simulink library "mobileRoboticsLib"  (R2017b)
settings: Solver=VariableStepAuto  StartTime=0.0  StopTime=10.0  RelTol=1e-3
undefined symbols (not defined in the file): b, DiscIntNeverNeededParam, r, X, Y, Z
libraries: sm_lib x67, nesl_utility x25, mobileRoboticsLib x11
(part 4 of 4)

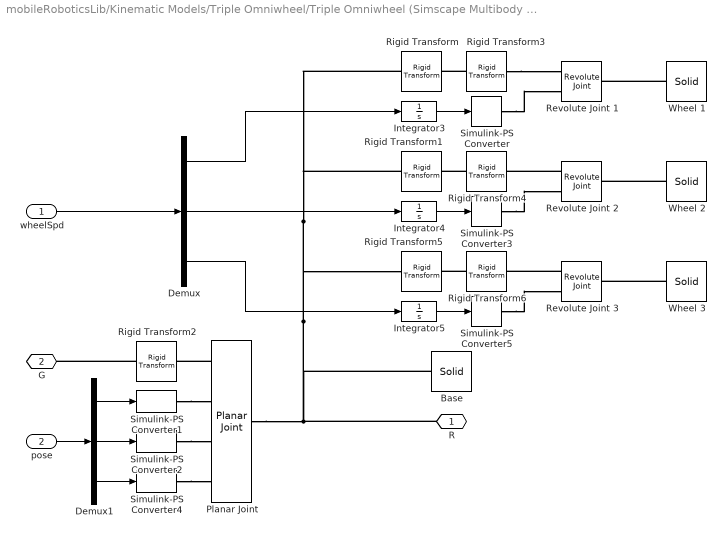
== system mobileRoboticsLib/Kinematic Models/Triple Omniwheel/Triple Omniwheel (Simscape Multibody Model) ==
  wheelSpd : Inport
  pose : Inport  Port=2
  Base : sm_lib/Body Elements/Solid  InertiaType=CalculateFromGeometry  Mass=chassisMass  MassUnits=kg  CenterOfMass=[0 0 0]  CenterOfMassUnits=m  MomentsOfInertia=[1 1 1]  MomentsOfInertiaUnits=kg*m^2  ProductsOfInertia=[1 1 1]  ProductsOfInertiaUnits=kg*m^2  DensityBased=on  Density=chassisMass  DensityUnits=kg/m^3  DoExposeReferenceFrame=on  SerializedFrames=<Frames/>  GraphicType=FromGeometry  MarkerShape=Sphere  MarkerSize=10  GraphicVisPropType=SimpleVisualProperties  GraphicDiffuseColor=chassisColor  GraphicSpecularColor=[0.5 0.5 0.5 1.0]  GraphicAmbientColor=[0.15 0.15 0.15 1.0]  GraphicEmissiveColor=[0.0 0.0 0.0 1.0]  GraphicShininess=75  GraphicOpacity=1.0  GeometryShape=Cylinder  RectangleSize=[1 1]  RectangleSizeUnits=m  BrickDimensions=[1 1 1]  BrickDimensionUnits=m  CylinderRadius=robotRadius-(wheelThickness/2)  CylinderRadiusUnits=m  CylinderLength=chassisThickness  CylinderLengthUnits=m  SphereRadius=1  SphereRadiusUnits=m  EllipsoidRadii=[1 1 1]  EllipsoidRadiiUnits=m  ExtrusionCrossSection=[1 1; -1 1; -1 -1; 1 -1]  ExtrusionCrossSectionUnits=m  ExtrusionLength=1  ExtrusionLengthUnits=m  PolygonNumSides=3  PolygonOuterRadius=1  PolygonOuterRadiusUnits=m  ExtGeomFileType=STEP  ExtGeomFileUnits=m  RevolutionCrossSection=[1 1; 1 -1; 2 -1; 2 1]  RevolutionCrossSectionUnits=m  RevolutionExtent=Full  RevolutionAngle=180  RevolutionAngleUnits=deg
  Demux : Demux  Outputs=3
  Demux1 : Demux  Outputs=3
  Integrator3 : Integrator
  Integrator4 : Integrator
  Integrator5 : Integrator
  Planar Joint : sm_lib/Joints/Planar Joint  SenseConstraintForce=off  SenseConstraintForceX=off  SenseConstraintForceY=off  SenseConstraintForceZ=off  SenseConstraintTorque=off  SenseConstraintTorqueX=off  SenseConstraintTorqueY=off  SenseConstraintTorqueZ=off  SenseTotalForce=off  SenseTotalForceX=off  SenseTotalForceY=off  SenseTotalForceZ=off  SenseTotalTorque=off  SenseTotalTorqueX=off  SenseTotalTorqueY=off  SenseTotalTorqueZ=off  CompositeWrenchDir=FollowerOnBase  CompositeWrenchFrame=BaseFrame  PxEquilibriumPosition=0  PxEquilibriumPositionUnits=m  PxSpringStiffness=0  PxSpringStiffnessUnits=N/m  PxDampingCoefficient=0  PxDampingCoefficientUnits=N/(m/s)  PxTorqueActuationMode=ComputedTorque  PxMotionActuationMode=InputMotion  PxSensePosition=off  PxSenseVelocity=off  PxSenseAcceleration=off  PxSenseTorqueForce=off  PxPositionTargetSpecify=on  PxPositionTargetPriority=High  PxPositionTargetValue=initX  PxPositionTargetValueUnits=m  PxVelocityTargetSpecify=off  PxVelocityTargetPriority=High  PxVelocityTargetValue=0  PxVelocityTargetValueUnits=m/s  PyEquilibriumPosition=0  PyEquilibriumPositionUnits=m  PySpringStiffness=0  PySpringStiffnessUnits=N/m  PyDampingCoefficient=0  PyDampingCoefficientUnits=N/(m/s)  PyTorqueActuationMode=ComputedTorque  PyMotionActuationMode=InputMotion  PySensePosition=off  PySenseVelocity=off  PySenseAcceleration=off  PySenseTorqueForce=off  PyPositionTargetSpecify=on  PyPositionTargetPriority=High  PyPositionTargetValue=initY  PyPositionTargetValueUnits=m  PyVelocityTargetSpecify=off  PyVelocityTargetPriority=High  PyVelocityTargetValue=0  PyVelocityTargetValueUnits=m/s  RzEquilibriumPosition=0  RzEquilibriumPositionUnits=deg  RzSpringStiffness=0  RzSpringStiffnessUnits=N*m/deg  RzDampingCoefficient=0  RzDampingCoefficientUnits=N*m/(deg/s)  RzTorqueActuationMode=ComputedTorque  RzMotionActuationMode=InputMotion  RzSensePosition=off  RzSenseVelocity=off  RzSenseAcceleration=off  RzSenseTorqueForce=off  RzPositionTargetSpecify=on  RzPositionTargetPriority=High  RzPositionTargetValue=initAngle  RzPositionTargetValueUnits=rad  RzVelocityTargetSpecify=off  RzVelocityTargetPriority=High  RzVelocityTargetValue=0  RzVelocityTargetValueUnits=deg/s
  Revolute Joint 1 : sm_lib/Joints/Revolute Joint  SenseConstraintForce=off  SenseConstraintForceX=off  SenseConstraintForceY=off  SenseConstraintForceZ=off  SenseConstraintTorque=off  SenseConstraintTorqueX=off  SenseConstraintTorqueY=off  SenseConstraintTorqueZ=off  SenseTotalForce=off  SenseTotalForceX=off  SenseTotalForceY=off  SenseTotalForceZ=off  SenseTotalTorque=off  SenseTotalTorqueX=off  SenseTotalTorqueY=off  SenseTotalTorqueZ=off  CompositeWrenchDir=FollowerOnBase  CompositeWrenchFrame=BaseFrame  EquilibriumPosition=0  EquilibriumPositionUnits=deg  SpringStiffness=0  SpringStiffnessUnits=N*m/deg  DampingCoefficient=0  DampingCoefficientUnits=N*m/(deg/s)  TorqueActuationMode=ComputedTorque  MotionActuationMode=InputMotion  SensePosition=off  SenseVelocity=off  SenseAcceleration=off  SenseTorqueForce=off  PositionTargetSpecify=off  PositionTargetPriority=High  PositionTargetValue=0  PositionTargetValueUnits=deg  VelocityTargetSpecify=off  VelocityTargetPriority=High  VelocityTargetValue=0  VelocityTargetValueUnits=deg/s
  Revolute Joint 2 : sm_lib/Joints/Revolute Joint  SenseConstraintForce=off  SenseConstraintForceX=off  SenseConstraintForceY=off  SenseConstraintForceZ=off  SenseConstraintTorque=off  SenseConstraintTorqueX=off  SenseConstraintTorqueY=off  SenseConstraintTorqueZ=off  SenseTotalForce=off  SenseTotalForceX=off  SenseTotalForceY=off  SenseTotalForceZ=off  SenseTotalTorque=off  SenseTotalTorqueX=off  SenseTotalTorqueY=off  SenseTotalTorqueZ=off  CompositeWrenchDir=FollowerOnBase  CompositeWrenchFrame=BaseFrame  EquilibriumPosition=0  EquilibriumPositionUnits=deg  SpringStiffness=0  SpringStiffnessUnits=N*m/deg  DampingCoefficient=0  DampingCoefficientUnits=N*m/(deg/s)  TorqueActuationMode=ComputedTorque  MotionActuationMode=InputMotion  SensePosition=off  SenseVelocity=off  SenseAcceleration=off  SenseTorqueForce=off  PositionTargetSpecify=off  PositionTargetPriority=High  PositionTargetValue=0  PositionTargetValueUnits=deg  VelocityTargetSpecify=off  VelocityTargetPriority=High  VelocityTargetValue=0  VelocityTargetValueUnits=deg/s
  Revolute Joint 3 : sm_lib/Joints/Revolute Joint  SenseConstraintForce=off  SenseConstraintForceX=off  SenseConstraintForceY=off  SenseConstraintForceZ=off  SenseConstraintTorque=off  SenseConstraintTorqueX=off  SenseConstraintTorqueY=off  SenseConstraintTorqueZ=off  SenseTotalForce=off  SenseTotalForceX=off  SenseTotalForceY=off  SenseTotalForceZ=off  SenseTotalTorque=off  SenseTotalTorqueX=off  SenseTotalTorqueY=off  SenseTotalTorqueZ=off  CompositeWrenchDir=FollowerOnBase  CompositeWrenchFrame=BaseFrame  EquilibriumPosition=0  EquilibriumPositionUnits=deg  SpringStiffness=0  SpringStiffnessUnits=N*m/deg  DampingCoefficient=0  DampingCoefficientUnits=N*m/(deg/s)  TorqueActuationMode=ComputedTorque  MotionActuationMode=InputMotion  SensePosition=off  SenseVelocity=off  SenseAcceleration=off  SenseTorqueForce=off  PositionTargetSpecify=off  PositionTargetPriority=High  PositionTargetValue=0  PositionTargetValueUnits=deg  VelocityTargetSpecify=off  VelocityTargetPriority=High  VelocityTargetValue=0  VelocityTargetValueUnits=deg/s
  Rigid Transform : sm_lib/Frames and Transforms/Rigid Transform  TranslationMethod=Cartesian  TranslationStandardOffset=0  TranslationLengthUnit=m  TranslationStandardAxis=+Y  TranslationCartesianOffset=[robotRadius*cos(wheelAngles(1)) robotRadius*sin(wheelAngles(1)) 0]  TranslationROffset=0  TranslationROffsetUnits=m  TranslationZOffset=0  TranslationZOffsetUnits=m  TranslationThetaOffset=0  TranslationThetaOffsetUnits=deg  RotationMethod=AlignedAxes  RotationAngleUnits=deg  RotationStandardAxis=+Z  RotationAngle=0.0  RotationArbitraryAxis=[0 0 1]  FollAlignAxisA=+Z  BaseAlignAxisA=+Y  FollAlignAxisB=+X  BaseAlignAxisB=+X  RotationSequenceAxes=FollowerAxes  RotationSequence=XYX  RotationSequenceAngles=[0 0 0]  RotationSequenceAnglesUnits=deg  RotationMatrix=[1 0 0; 0 1 0; 0 0 1]
  Rigid Transform1 : sm_lib/Frames and Transforms/Rigid Transform  TranslationMethod=Cartesian  TranslationStandardOffset=0  TranslationLengthUnit=m  TranslationStandardAxis=+Y  TranslationCartesianOffset=[robotRadius*cos(wheelAngles(2)) robotRadius*sin(wheelAngles(2)) 0]  TranslationROffset=0  TranslationROffsetUnits=m  TranslationZOffset=0  TranslationZOffsetUnits=m  TranslationThetaOffset=0  TranslationThetaOffsetUnits=deg  RotationMethod=AlignedAxes  RotationAngleUnits=deg  RotationStandardAxis=+Z  RotationAngle=0.0  RotationArbitraryAxis=[0 0 1]  FollAlignAxisA=+Z  BaseAlignAxisA=+Y  FollAlignAxisB=+X  BaseAlignAxisB=+X  RotationSequenceAxes=FollowerAxes  RotationSequence=XYX  RotationSequenceAngles=[0 0 0]  RotationSequenceAnglesUnits=deg  RotationMatrix=[1 0 0; 0 1 0; 0 0 1]
  Rigid Transform2 : sm_lib/Frames and Transforms/Rigid Transform  TranslationMethod=StandardAxis  TranslationStandardOffset=wheelRadius  TranslationLengthUnit=m  TranslationStandardAxis=+Z  TranslationCartesianOffset=[0 0 0]  TranslationROffset=0  TranslationROffsetUnits=m  TranslationZOffset=0  TranslationZOffsetUnits=m  TranslationThetaOffset=0  TranslationThetaOffsetUnits=deg  RotationMethod=None  RotationAngleUnits=deg  RotationStandardAxis=+Z  RotationAngle=0.0  RotationArbitraryAxis=[0 0 1]  FollAlignAxisA=+Z  BaseAlignAxisA=+Y  FollAlignAxisB=+X  BaseAlignAxisB=+X  RotationSequenceAxes=FollowerAxes  RotationSequence=XYX  RotationSequenceAngles=[0 0 0]  RotationSequenceAnglesUnits=deg  RotationMatrix=[1 0 0; 0 1 0; 0 0 1]
  Rigid Transform3 : sm_lib/Frames and Transforms/Rigid Transform  TranslationMethod=None  TranslationStandardOffset=0  TranslationLengthUnit=m  TranslationStandardAxis=+Z  TranslationCartesianOffset=[0 0 0]  TranslationROffset=0  TranslationROffsetUnits=m  TranslationZOffset=0  TranslationZOffsetUnits=m  TranslationThetaOffset=0  TranslationThetaOffsetUnits=deg  RotationMethod=StandardAxis  RotationAngleUnits=rad  RotationStandardAxis=+Y  RotationAngle=pi/2-wheelAngles(1)  RotationArbitraryAxis=[0 0 1]  FollAlignAxisA=+X  BaseAlignAxisA=+Y  FollAlignAxisB=+Y  BaseAlignAxisB=+Z  RotationSequenceAxes=FollowerAxes  RotationSequence=XYX  RotationSequenceAngles=[0 0 0]  RotationSequenceAnglesUnits=deg  RotationMatrix=[1 0 0; 0 1 0; 0 0 1]
  Rigid Transform4 : sm_lib/Frames and Transforms/Rigid Transform  TranslationMethod=None  TranslationStandardOffset=0  TranslationLengthUnit=m  TranslationStandardAxis=+Z  TranslationCartesianOffset=[0 0 0]  TranslationROffset=0  TranslationROffsetUnits=m  TranslationZOffset=0  TranslationZOffsetUnits=m  TranslationThetaOffset=0  TranslationThetaOffsetUnits=deg  RotationMethod=StandardAxis  RotationAngleUnits=rad  RotationStandardAxis=+Y  RotationAngle=pi/2-wheelAngles(2)  RotationArbitraryAxis=[0 0 1]  FollAlignAxisA=+X  BaseAlignAxisA=+Y  FollAlignAxisB=+Y  BaseAlignAxisB=+Z  RotationSequenceAxes=FollowerAxes  RotationSequence=XYX  RotationSequenceAngles=[0 0 0]  RotationSequenceAnglesUnits=deg  RotationMatrix=[1 0 0; 0 1 0; 0 0 1]
  Rigid Transform5 : sm_lib/Frames and Transforms/Rigid Transform  TranslationMethod=Cartesian  TranslationStandardOffset=0  TranslationLengthUnit=m  TranslationStandardAxis=+Y  TranslationCartesianOffset=[robotRadius*cos(wheelAngles(3)) robotRadius*sin(wheelAngles(3)) 0]  TranslationROffset=0  TranslationROffsetUnits=m  TranslationZOffset=0  TranslationZOffsetUnits=m  TranslationThetaOffset=0  TranslationThetaOffsetUnits=deg  RotationMethod=AlignedAxes  RotationAngleUnits=deg  RotationStandardAxis=+Z  RotationAngle=0.0  RotationArbitraryAxis=[0 0 1]  FollAlignAxisA=+Z  BaseAlignAxisA=+Y  FollAlignAxisB=+X  BaseAlignAxisB=+X  RotationSequenceAxes=FollowerAxes  RotationSequence=XYX  RotationSequenceAngles=[0 0 0]  RotationSequenceAnglesUnits=deg  RotationMatrix=[1 0 0; 0 1 0; 0 0 1]
  Rigid Transform6 : sm_lib/Frames and Transforms/Rigid Transform  TranslationMethod=None  TranslationStandardOffset=0  TranslationLengthUnit=m  TranslationStandardAxis=+Z  TranslationCartesianOffset=[0 0 0]  TranslationROffset=0  TranslationROffsetUnits=m  TranslationZOffset=0  TranslationZOffsetUnits=m  TranslationThetaOffset=0  TranslationThetaOffsetUnits=deg  RotationMethod=StandardAxis  RotationAngleUnits=rad  RotationStandardAxis=+Y  RotationAngle=pi/2-wheelAngles(3)  RotationArbitraryAxis=[0 0 1]  FollAlignAxisA=+X  BaseAlignAxisA=+Y  FollAlignAxisB=+Y  BaseAlignAxisB=+Z  RotationSequenceAxes=FollowerAxes  RotationSequence=XYX  RotationSequenceAngles=[0 0 0]  RotationSequenceAnglesUnits=deg  RotationMatrix=[1 0 0; 0 1 0; 0 0 1]
  Simulink-PS Converter{,1..5} (6 alike) : nesl_utility/Simulink-PS Converter  PhysicalDomain=network_engine_domain  SubClassName=ps_input  LeftPortType=input  RightPortType=output  PseudoPeriodic=off  Frequencies=[]  NoiseDistribution=none  NoiseParameters=[]  Unit=1  AffineConversion=off  FilteringAndDerivatives=filter  SimscapeFilterOrder=2  InputFilterTimeConstant=timeConstant  UdotUserProvided=0
  Wheel 1 : sm_lib/Body Elements/Solid  InertiaType=CalculateFromGeometry  Mass=wheelMass  MassUnits=kg  CenterOfMass=[0 0 0]  CenterOfMassUnits=m  MomentsOfInertia=[1 1 1]  MomentsOfInertiaUnits=kg*m^2  ProductsOfInertia=[1 1 1]  ProductsOfInertiaUnits=kg*m^2  DensityBased=on  Density=1000  DensityUnits=kg/m^3  DoExposeReferenceFrame=on  SerializedFrames=<Frames/>  GraphicType=FromGeometry  MarkerShape=Sphere  MarkerSize=10  GraphicVisPropType=SimpleVisualProperties  GraphicDiffuseColor=wheelColor  GraphicSpecularColor=[0.5 0.5 0.5 1.0]  GraphicAmbientColor=[0.15 0.15 0.15 1.0]  GraphicEmissiveColor=[0.0 0.0 0.0 1.0]  GraphicShininess=75  GraphicOpacity=1.0  GeometryShape=Cylinder  RectangleSize=[1 1]  RectangleSizeUnits=m  BrickDimensions=[1 1 1]  BrickDimensionUnits=m  CylinderRadius=wheelRadius  CylinderRadiusUnits=m  CylinderLength=wheelThickness  CylinderLengthUnits=m  SphereRadius=1  SphereRadiusUnits=m  EllipsoidRadii=[1 1 1]  EllipsoidRadiiUnits=m  ExtrusionCrossSection=[1 1; -1 1; -1 -1; 1 -1]  ExtrusionCrossSectionUnits=m  ExtrusionLength=1  ExtrusionLengthUnits=m  PolygonNumSides=3  PolygonOuterRadius=1  PolygonOuterRadiusUnits=m  ExtGeomFileType=STEP  ExtGeomFileUnits=m  RevolutionCrossSection=[1 1; 1 -1; 2 -1; 2 1]  RevolutionCrossSectionUnits=m  RevolutionExtent=Full  RevolutionAngle=180  RevolutionAngleUnits=deg
  Wheel 2 : sm_lib/Body Elements/Solid  InertiaType=CalculateFromGeometry  Mass=wheelMass  MassUnits=kg  CenterOfMass=[0 0 0]  CenterOfMassUnits=m  MomentsOfInertia=[1 1 1]  MomentsOfInertiaUnits=kg*m^2  ProductsOfInertia=[1 1 1]  ProductsOfInertiaUnits=kg*m^2  DensityBased=on  Density=1000  DensityUnits=kg/m^3  DoExposeReferenceFrame=on  SerializedFrames=<Frames/>  GraphicType=FromGeometry  MarkerShape=Sphere  MarkerSize=10  GraphicVisPropType=SimpleVisualProperties  GraphicDiffuseColor=wheelColor  GraphicSpecularColor=[0.5 0.5 0.5 1.0]  GraphicAmbientColor=[0.15 0.15 0.15 1.0]  GraphicEmissiveColor=[0.0 0.0 0.0 1.0]  GraphicShininess=75  GraphicOpacity=1.0  GeometryShape=Cylinder  RectangleSize=[1 1]  RectangleSizeUnits=m  BrickDimensions=[1 1 1]  BrickDimensionUnits=m  CylinderRadius=wheelRadius  CylinderRadiusUnits=m  CylinderLength=wheelThickness  CylinderLengthUnits=m  SphereRadius=1  SphereRadiusUnits=m  EllipsoidRadii=[1 1 1]  EllipsoidRadiiUnits=m  ExtrusionCrossSection=[1 1; -1 1; -1 -1; 1 -1]  ExtrusionCrossSectionUnits=m  ExtrusionLength=1  ExtrusionLengthUnits=m  PolygonNumSides=3  PolygonOuterRadius=1  PolygonOuterRadiusUnits=m  ExtGeomFileType=STEP  ExtGeomFileUnits=m  RevolutionCrossSection=[1 1; 1 -1; 2 -1; 2 1]  RevolutionCrossSectionUnits=m  RevolutionExtent=Full  RevolutionAngle=180  RevolutionAngleUnits=deg
  Wheel 3 : sm_lib/Body Elements/Solid  InertiaType=CalculateFromGeometry  Mass=wheelMass  MassUnits=kg  CenterOfMass=[0 0 0]  CenterOfMassUnits=m  MomentsOfInertia=[1 1 1]  MomentsOfInertiaUnits=kg*m^2  ProductsOfInertia=[1 1 1]  ProductsOfInertiaUnits=kg*m^2  DensityBased=on  Density=1000  DensityUnits=kg/m^3  DoExposeReferenceFrame=on  SerializedFrames=<Frames/>  GraphicType=FromGeometry  MarkerShape=Sphere  MarkerSize=10  GraphicVisPropType=SimpleVisualProperties  GraphicDiffuseColor=wheelColor  GraphicSpecularColor=[0.5 0.5 0.5 1.0]  GraphicAmbientColor=[0.15 0.15 0.15 1.0]  GraphicEmissiveColor=[0.0 0.0 0.0 1.0]  GraphicShininess=75  GraphicOpacity=1.0  GeometryShape=Cylinder  RectangleSize=[1 1]  RectangleSizeUnits=m  BrickDimensions=[1 1 1]  BrickDimensionUnits=m  CylinderRadius=wheelRadius  CylinderRadiusUnits=m  CylinderLength=wheelThickness  CylinderLengthUnits=m  SphereRadius=1  SphereRadiusUnits=m  EllipsoidRadii=[1 1 1]  EllipsoidRadiiUnits=m  ExtrusionCrossSection=[1 1; -1 1; -1 -1; 1 -1]  ExtrusionCrossSectionUnits=m  ExtrusionLength=1  ExtrusionLengthUnits=m  PolygonNumSides=3  PolygonOuterRadius=1  PolygonOuterRadiusUnits=m  ExtGeomFileType=STEP  ExtGeomFileUnits=m  RevolutionCrossSection=[1 1; 1 -1; 2 -1; 2 1]  RevolutionCrossSectionUnits=m  RevolutionExtent=Full  RevolutionAngle=180  RevolutionAngleUnits=deg
  R : PMIOPort  Port=1  Side=Right
  G : PMIOPort  Port=2  Side=Right
  wires:
  wheelSpd/1 -> Demux/1
  Demux1/1 -> Simulink-PS Converter1/1
  Demux1/2 -> Simulink-PS Converter2/1
  Demux1/3 -> Simulink-PS Converter4/1
  pose/1 -> Demux1/1
  Integrator5/1 -> Simulink-PS Converter5/1
  Integrator3/1 -> Simulink-PS Converter/1
  Integrator4/1 -> Simulink-PS Converter3/1
  Demux/1 -> Integrator3/1
  Demux/2 -> Integrator4/1
  Demux/3 -> Integrator5/1
  connections:
  Simulink-PS Converter1/RConn1 -- Planar Joint/LConn2
  Rigid Transform2/LConn1 -- G/RConn1
  Simulink-PS Converter4/RConn1 -- Planar Joint/LConn4
  Simulink-PS Converter2/RConn1 -- Planar Joint/LConn3
  Planar Joint/LConn1 -- Rigid Transform2/RConn1
  R/RConn1 -- Planar Joint/RConn1 -- Base/RConn1 -- Rigid Transform/LConn1 -- Rigid Transform1/LConn1 -- Rigid Transform5/LConn1
  Rigid Transform6/LConn1 -- Rigid Transform5/RConn1
  Rigid Transform3/RConn1 -- Revolute Joint 1/LConn1
  Revolute Joint 3/LConn1 -- Rigid Transform6/RConn1
  Revolute Joint 2/LConn1 -- Rigid Transform4/RConn1
  Simulink-PS Converter3/RConn1 -- Revolute Joint 2/LConn2
  Simulink-PS Converter5/RConn1 -- Revolute Joint 3/LConn2
  Wheel 1/RConn1 -- Revolute Joint 1/RConn1
  Rigid Transform3/LConn1 -- Rigid Transform/RConn1
  Simulink-PS Converter/RConn1 -- Revolute Joint 1/LConn2
  Wheel 2/RConn1 -- Revolute Joint 2/RConn1
  Rigid Transform4/LConn1 -- Rigid Transform1/RConn1
  Wheel 3/RConn1 -- Revolute Joint 3/RConn1

== system mobileRoboticsLib/Kinematic Models/Triple Omniwheel/Triple Omniwheel Forward Kinematics ==
  wheelSpd : Inport
  MATLAB Function : MATLAB Function  TreatAsAtomicUnit=on
  bodySpd : Outport
  wires:
  wheelSpd/1 -> MATLAB Function/1(wheelSpeeds)  "wheelSpeeds"
  MATLAB Function/1(bodySpeed) -> bodySpd/1  "bodySpeed"

== system mobileRoboticsLib/Kinematic Models/Triple Omniwheel/Triple Omniwheel Inverse Kinematics  ==
  vRef : Inport
  MATLAB Function : MATLAB Function  TreatAsAtomicUnit=on
  wheelSpd : Outport
  wires:
  MATLAB Function/1(wheelSpeeds) -> wheelSpd/1  "wheelSpeeds"
  vRef/1 -> MATLAB Function/1(bodySpeed)  "bodySpeed"

== system mobileRoboticsLib/Kinematic Models/Triple Omniwheel/Triple Omniwheel Simulation ==
  wheelSpd : Inport
  Generic Robot Simulation : mobileRoboticsLib/Utilities/Generic Vehicle Simulation  initX=initX  initY=initY  initAngle=initAngle  Ts=Ts
      settings: SourceProductName=Mobile Robotics Simulation Toolbox
  Triple Omniwheel Forward Kinematics : mobileRoboticsLib/Kinematic Models/Triple Omniwheel/Triple Omniwheel Forward Kinematics  wheelRadius=wheelRadius  robotRadius=robotRadius  wheelAngles=wheelAngles
      settings: SourceProductName=Mobile Robotics Simulation Toolbox
  pose : Outport
  wires:
  wheelSpd/1 -> Triple Omniwheel Forward Kinematics/1
  Triple Omniwheel Forward Kinematics/1 -> Generic Robot Simulation/1
  Generic Robot Simulation/1 -> pose/1

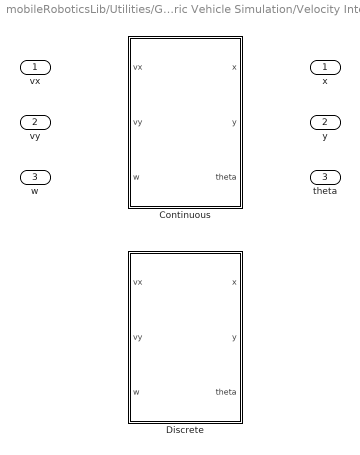
== system mobileRoboticsLib/Utilities/Generic Vehicle Simulation/Velocity Integrator ==
  "vx " : Inport
  "vy " : Inport  Port=2
  "w " : Inport  Port=3
  Continuous : Subsystem  VariantControl=mode==1
  Discrete : Subsystem  VariantControl=mode==2
  " x" : Outport
  " y" : Outport  Port=2
  " theta" : Outport  Port=3

== system mobileRoboticsLib/Kinematic Models/Four-Wheel Steering/Four-Wheel Steering Inverse Kinematics/Inverse Kinematics ==
  ref : Inport
  Front Steering : MATLAB Function  TreatAsAtomicUnit=on  VariantControl=mode==1
  Parallel Steering : MATLAB Function  TreatAsAtomicUnit=on  VariantControl=mode==2
  Zero Sideslip : MATLAB Function  TreatAsAtomicUnit=on  VariantControl=mode==3
  " wheelSpeeds" : Outport
  " steerAngles" : Outport  Port=2

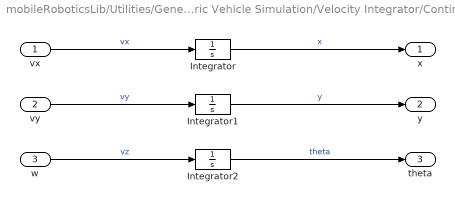
== system mobileRoboticsLib/Utilities/Generic Vehicle Simulation/Velocity Integrator/Continuous ==
  vx : Inport
  vy : Inport  Port=2
  w : Inport  Port=3
  Integrator : Integrator  InitialCondition=initX
  Integrator1 : Integrator  InitialCondition=initY
  Integrator2 : Integrator  InitialCondition=initAngle
  x : Outport
  y : Outport  Port=2
  theta : Outport  Port=3
  wires:
  Integrator1/1 -> y/1  "y"
  vy/1 -> Integrator1/1  "vy"
  Integrator/1 -> x/1  "x"
  vx/1 -> Integrator/1  "vx"
  w/1 -> Integrator2/1  "vz"
  Integrator2/1 -> theta/1  "theta"

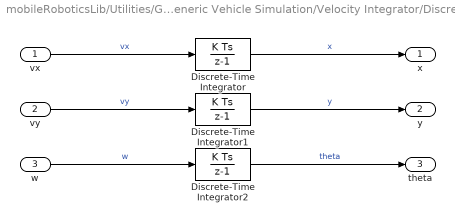
== system mobileRoboticsLib/Utilities/Generic Vehicle Simulation/Velocity Integrator/Discrete ==
  vx : Inport
  vy : Inport  Port=2
  w : Inport  Port=3
  Discrete-Time Integrator : DiscreteIntegrator  InitialCondition=initX  InitialConditionSetting=State (most efficient)  SampleTime=Ts  ICPrevOutput=DiscIntNeverNeededParam  ICPrevScaledInput=DiscIntNeverNeededParam
  Discrete-Time Integrator1 : DiscreteIntegrator  InitialCondition=initY  InitialConditionSetting=State (most efficient)  SampleTime=Ts  ICPrevOutput=DiscIntNeverNeededParam  ICPrevScaledInput=DiscIntNeverNeededParam
  Discrete-Time Integrator2 : DiscreteIntegrator  InitialCondition=initAngle  InitialConditionSetting=State (most efficient)  SampleTime=Ts  ICPrevOutput=DiscIntNeverNeededParam  ICPrevScaledInput=DiscIntNeverNeededParam
  x : Outport
  y : Outport  Port=2
  theta : Outport  Port=3
  wires:
  Discrete-Time Integrator2/1 -> theta/1  "theta"
  w/1 -> Discrete-Time Integrator2/1  "w"
  vx/1 -> Discrete-Time Integrator/1  "vx"
  Discrete-Time Integrator/1 -> x/1  "x"
  vy/1 -> Discrete-Time Integrator1/1  "vy"
  Discrete-Time Integrator1/1 -> y/1  "y"

== matlab function mobileRoboticsLib/Kinematic Models/Differential Drive/Differential Drive Forward Kinematics/MATLAB Function ==
  settings: updateMethod=DISCRETE
  data: wL input; v output; wR input; wheelBase parameter; w output; wheelRadius parameter
function [v,w] = diffDriveFwdKin(wL,wR,wheelBase, wheelRadius)
    
    % Initialize DifferentialDrive object
    persistent robot
    if isempty(robot)
        robot = DifferentialDrive(wheelRadius,wheelBase);
    end
    
    % Run object's forward kinematics method
    [v,w] = forwardKinematics(robot,wL,wR);

end

== matlab function mobileRoboticsLib/Kinematic Models/Differential Drive/Differential Drive Inverse Kinematics/MATLAB Function ==
  data: v input; wL output; w input; wR output; wheelRadius parameter; wheelBase parameter
function [wL,wR] = diffDriveInvKin(v,w,wheelRadius,wheelBase)
    
    % Initialize DifferentialDrive object
    persistent robot
    if isempty(robot)
        robot = DifferentialDrive(wheelRadius,wheelBase);
    end
    
    % Run object's forward kinematics method
    [wL,wR] = inverseKinematics(robot,v,w);

end

== matlab function mobileRoboticsLib/Kinematic Models/Four-Wheel Steering/Four-Wheel Steering Forward Kinematics/MATLAB Function ==
  settings: updateMethod=DISCRETE
  data: wheelSpeeds input; bodySpeed output; wheelRadius parameter; frontWheelDist parameter; rearWheelDist parameter; steerAngles input
function bodySpeed = fourWheelSteerFwdKin(wheelSpeeds,wheelRadius,frontWheelDist,rearWheelDist, steerAngles) ...
    
    % Initialize Four-Wheel Steering object
    persistent robot
    if isempty(robot)
        robot = FourWheelSteering(wheelRadius,[frontWheelDist,rearWheelDist]);
    end
    
    % Run object's forward kinematics method
    bodySpeed = forwardKinematics(robot,wheelSpeeds,steerAngles);

end

== matlab function mobileRoboticsLib/Kinematic Models/Triple Omniwheel/Triple Omniwheel Inverse Kinematics /MATLAB Function ==
  data: bodySpeed input; wheelRadius parameter; wheelSpeeds output size=3; wheelAngles parameter; robotRadius parameter
function wheelSpeeds = tripleOmniInverseKinematics(bodySpeed,wheelRadius,wheelAngles, robotRadius)
    
    % Initialize TripleOmniwheel object
    persistent robot
    if isempty(robot)
        robot = TripleOmniwheel(wheelRadius,robotRadius,wheelAngles);
    end
    
    % Run object's inverse kinematics method
    wheelSpeeds = inverseKinematics(robot,bodySpeed);

end

== matlab function mobileRoboticsLib/Kinematic Models/Four-Wheel Steering/Four-Wheel Steering Inverse Kinematics/Inverse Kinematics/Front Steering ==
  data: ref input; wheelRadius parameter; wheelSpeeds output; frontWheelDist parameter; rearWheelDist parameter; steerAngles output
function [wheelSpeeds,steerAngles] = fourWheelSteerInvKinFrontSteer ...
         (ref,wheelRadius,frontWheelDist,rearWheelDist)
    % ref = [vx;w]
    
    % Initialize FourWheelSteering object
    persistent robot
    if isempty(robot)
        robot = FourWheelSteering(wheelRadius,[frontWheelDist,rearWheelDist]);
    end
    
    % Run object's inverse kinematics method
    [wheelSpeeds,steerAngles] = ...
        inverseKinematicsFrontSteer(robot,ref(1),ref(2));

end

== matlab function mobileRoboticsLib/Kinematic Models/Triple Omniwheel/Triple Omniwheel Forward Kinematics/MATLAB Function ==
  settings: updateMethod=DISCRETE
  data: wheelSpeeds input; bodySpeed output; wheelRadius parameter; robotRadius parameter; wheelAngles parameter
function bodySpeed = tripleOmniFwdKin(wheelSpeeds,wheelRadius,robotRadius,wheelAngles)
    
    % Initialize TripleOmniwheel object
    persistent robot
    if isempty(robot)
        robot = TripleOmniwheel(wheelRadius,robotRadius,wheelAngles);
    end
    
    % Run object's forward kinematics method
    bodySpeed = forwardKinematics(robot,wheelSpeeds);

end

== matlab function mobileRoboticsLib/Kinematic Models/Four-Wheel Steering/Four-Wheel Steering Inverse Kinematics/Inverse Kinematics/Zero Sideslip ==
  data: ref input; wheelRadius parameter; wheelSpeeds output; frontWheelDist parameter; rearWheelDist parameter; steerAngles output
function [wheelSpeeds,steerAngles] = fourWheelSteerInvKinZeroSideslip ...
         (ref,wheelRadius,frontWheelDist,rearWheelDist)
    % ref = [vx;w]

    % Initialize FourWheelSteering object
    persistent robot
    if isempty(robot)
        robot = FourWheelSteering(wheelRadius,[frontWheelDist,rearWheelDist]);
    end
    
    % Run object's inverse kinematics method
    [wheelSpeeds,steerAngles] = ... 
        inverseKinematicsZeroSideslip(robot,ref(1),ref(2));

end

== matlab function mobileRoboticsLib/Kinematic Models/Four-Wheel Steering/Four-Wheel Steering Inverse Kinematics/Inverse Kinematics/Parallel Steering ==
  data: ref input; wheelRadius parameter; wheelSpeeds output; frontWheelDist parameter; rearWheelDist parameter; steerAngles output
function [wheelSpeeds,steerAngles] = fourWheelSteerInvKinParallelSteer ...
         (ref,wheelRadius,frontWheelDist,rearWheelDist)
    % ref = [vx;vy]
    
    % Initialize FourWheelSteering object
    persistent robot
    if isempty(robot)
        robot = FourWheelSteering(wheelRadius,[frontWheelDist,rearWheelDist]);
    end
    
    % Run object's inverse kinematics method
    [wheelSpeeds,steerAngles] = ... 
        inverseKinematicsParallelSteer(robot,ref(1),ref(2));

end

== matlab function mobileRoboticsLib/Kinematic Models/Four-Wheel Mecanum/Four-Wheel Mecanum Forward Kinematics/MATLAB Function ==
  settings: updateMethod=DISCRETE
  data: wheelSpeeds input; bodySpeed output; wheelRadius parameter; wheelBase parameter; wheelTrack parameter
function bodySpeed = fourWheelMecanumFwdKin(wheelSpeeds,wheelRadius,wheelBase,wheelTrack)
    
    % Initialize FourWheelMecanum object
    persistent robot
    if isempty(robot)
        robot = FourWheelMecanum(wheelRadius,wheelBase,wheelTrack);
    end
    
    % Run object's forward kinematics method
    bodySpeed = forwardKinematics(robot,wheelSpeeds);

end

== matlab function mobileRoboticsLib/Kinematic Models/Four-Wheel Mecanum/Four-Wheel Mecanum Inverse Kinematics/MATLAB Function ==
  data: bodySpeed input; wheelRadius parameter; wheelSpeeds output; wheelBase parameter; wheelTrack parameter
function wheelSpeeds = fourWheelMecanumInvKin(bodySpeed,wheelRadius,wheelBase,wheelTrack)
    
    % Initialize FourWheelMecanum object
    persistent robot
    if isempty(robot)
        robot = FourWheelMecanum(wheelRadius,wheelBase,wheelTrack);
    end
    
    % Run object's inverse kinematics method
    wheelSpeeds = inverseKinematics(robot,bodySpeed);

end

== matlab function mobileRoboticsLib/Environments/Multi-Robot Environment/MATLAB Function ==
  data: wps input; objs input
function visualizeWaypointsAndObjects(wps,objs)

    coder.extrinsic('internal.multiRobotVizWorld')
    internal.multiRobotVizWorld(wps,objs)

end

== matlab function mobileRoboticsLib/Environments/Multi-Robot Visualizer/MATLAB Function ==
  data: pose input; rngs input; idx parameter; hasLidar parameter
function visualizeRobot(pose, rngs, idx, hasLidar)

    coder.extrinsic('internal.multiRobotVizSet');
    if hasLidar
        internal.multiRobotVizSet(idx,pose,rngs);
    else
        internal.multiRobotVizSet(idx,pose,[]);
    end

end

== matlab function mobileRoboticsLib/Kinematic Models/Generic Omniwheel/Generic Omniwheel Forward Kinematics/MATLAB Function ==
  settings: updateMethod=DISCRETE
  data: wheelSpeeds input; bodySpeed output; wheelRadius parameter; wheelPositions parameter; wheelAngles parameter
function bodySpeed = genericOmniFwdKin(wheelSpeeds,wheelRadius,wheelPositions,wheelAngles)
    
    % Initialize TripleOmniwheel object
    persistent robot
    if isempty(robot)
        robot = GenericOmniwheel(wheelRadius,wheelPositions,wheelAngles);
    end
    
    % Run object's forward kinematics method
    bodySpeed = forwardKinematics(robot,wheelSpeeds);

end

== matlab function mobileRoboticsLib/Kinematic Models/Generic Omniwheel/Generic Omniwheel Inverse Kinematics /MATLAB Function ==
  data: bodySpeed input; wheelRadius parameter; wheelPositions parameter; wheelSpeeds output; wheelAngles parameter
function wheelSpeeds = genericOmniInverseKinematics(bodySpeed,wheelRadius,wheelPositions,wheelAngles)
    
    % Initialize TripleOmniwheel object
    persistent robot
    if isempty(robot)
        robot = GenericOmniwheel(wheelRadius,wheelPositions,wheelAngles);
    end
    
    % Run object's inverse kinematics method
    wheelSpeeds = inverseKinematics(robot,bodySpeed);

end
